simulink model "CTRL_SPECCTRL_FB_STRAT1_YAWM_test"  (R2024b)
settings: Solver=VariableStepAuto  StartTime=0.0  StopTime=10.0  RelTol=1e-3
libraries: CTRL_SPECCTRL_FB_STRAT1_YAWM x1
settings Model: Creator=blatak  LastModifiedBy=blatak

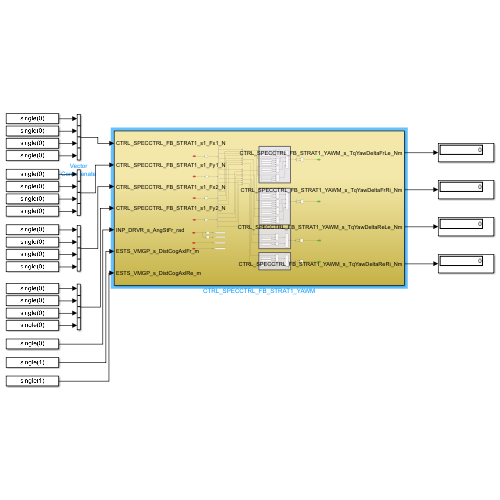
[thumbnail: Simulink's stored preview of the top-level diagram]
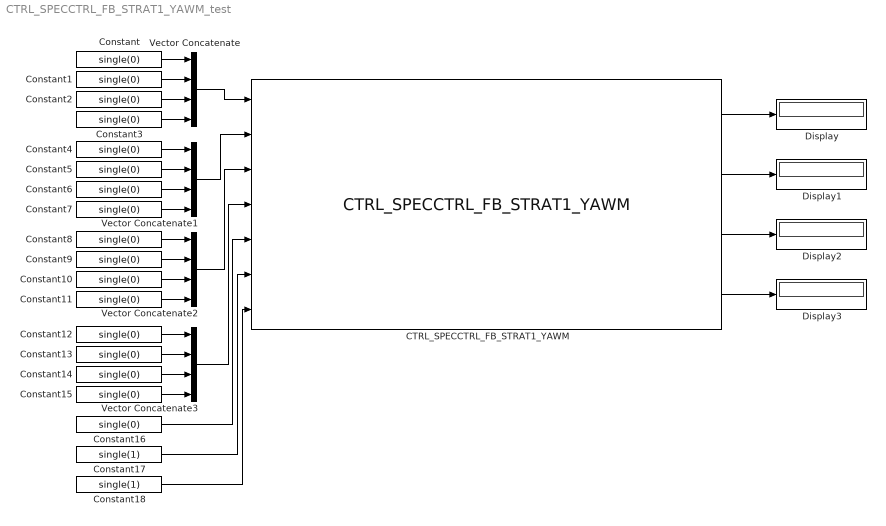
== system CTRL_SPECCTRL_FB_STRAT1_YAWM_test ==
  CTRL_SPECCTRL_FB_STRAT1_YAWM : CTRL_SPECCTRL_FB_STRAT1_YAWM/CTRL_SPECCTRL_FB_STRAT1_YAWM  SystemSampleTime=-1  VariantActivationTime=update diagram  AllowFlexibleInterface=on  Latency=0  AutoFrameSizeCalculation=off
  Constant{,1..16} (17 alike) : Constant  Value=single(0)
  Constant17 : Constant  Value=single(1)
  Constant18 : Constant  Value=single(1)
  Display{,1..3} (4 alike) : Display
  Vector Concatenate{,1..3} (4 alike) : Concatenate  NumInputs=4
  wires:
  Constant/1 -> Vector Concatenate/1
  Constant1/1 -> Vector Concatenate/2
  Constant2/1 -> Vector Concatenate/3
  Constant3/1 -> Vector Concatenate/4
  Constant4/1 -> Vector Concatenate1/1
  Constant5/1 -> Vector Concatenate1/2
  Constant6/1 -> Vector Concatenate1/3
  Constant7/1 -> Vector Concatenate1/4
  Constant8/1 -> Vector Concatenate2/1
  Constant9/1 -> Vector Concatenate2/2
  Constant10/1 -> Vector Concatenate2/3
  Constant11/1 -> Vector Concatenate2/4
  Constant12/1 -> Vector Concatenate3/1
  Constant13/1 -> Vector Concatenate3/2
  Constant14/1 -> Vector Concatenate3/3
  Constant15/1 -> Vector Concatenate3/4
  Constant18/1 -> CTRL_SPECCTRL_FB_STRAT1_YAWM/7
  Constant17/1 -> CTRL_SPECCTRL_FB_STRAT1_YAWM/6
  Constant16/1 -> CTRL_SPECCTRL_FB_STRAT1_YAWM/5
  Vector Concatenate3/1 -> CTRL_SPECCTRL_FB_STRAT1_YAWM/4
  Vector Concatenate2/1 -> CTRL_SPECCTRL_FB_STRAT1_YAWM/3
  Vector Concatenate1/1 -> CTRL_SPECCTRL_FB_STRAT1_YAWM/2
  Vector Concatenate/1 -> CTRL_SPECCTRL_FB_STRAT1_YAWM/1
  CTRL_SPECCTRL_FB_STRAT1_YAWM/1 -> Display/1
  CTRL_SPECCTRL_FB_STRAT1_YAWM/2 -> Display1/1
  CTRL_SPECCTRL_FB_STRAT1_YAWM/3 -> Display2/1
  CTRL_SPECCTRL_FB_STRAT1_YAWM/4 -> Display3/1
